simulink model "exampleModel_bus_axi_w_4ptavg"  (R2017b)
settings: Solver=VariableStepAuto  StartTime=0.0  StopTime=10e-5  RelTol=1e-3
PreLoadFcn:
  | setup
values from neighbouring files (symbols this model uses):
  axiClk = 156.25e6    (= 156250000)    [setup.m]    (also in setup_exampleModel_bus_axi_simulink.m; setup_exampleModel_bus_axi_simulink_lcls2.m; setup_lcls2_pcav.m; sysgen_signal.m)
  cav1p1_addr = 204    [setup_exampleModel_bus_axi_simulink.m]    (also in setup_exampleModel_bus_axi_simulink_lcls2.m; setup_lcls2_pcav.m; sysgen_signal.m)
  cav1p2_addr = cav1p1_addr * 2    (= 408)    [setup_exampleModel_bus_axi_simulink.m]    (also in setup_exampleModel_bus_axi_simulink_lcls2.m; setup_lcls2_pcav.m; sysgen_signal.m)
  cav2p1_addr = cav1p1_addr * 3    (= 612)    [setup_exampleModel_bus_axi_simulink.m]    (also in setup_exampleModel_bus_axi_simulink_lcls2.m; setup_lcls2_pcav.m; sysgen_signal.m)
  cav2p2_addr = cav1p1_addr * 4    (= 816)    [setup_exampleModel_bus_axi_simulink.m]    (also in setup_exampleModel_bus_axi_simulink_lcls2.m; setup_lcls2_pcav.m; sysgen_signal.m)
  Fadc = Fs/interleavedChannels    (= 29750000)    [setup.m]    (also in setup_exampleModel_bus_axi_simulink.m = 357000000; setup_exampleModel_bus_axi_simulink_lcls2.m = 351000000; setup_lcls2_pcav.m = 357000000; sysgen_signal.m = 357000000)
  fir_lpf = fir1(15, w_lpf)    [setup_exampleModel_bus_axi_simulink.m]    (also in setup_exampleModel_bus_axi_simulink_lcls2.m; setup_lcls2_pcav.m)
  Fproc = 204e6    (= 204000000)    [setup_exampleModel_bus_axi_simulink.m]    (also in setup_exampleModel_bus_axi_simulink_lcls2.m = 200571400; setup_lcls2_pcav.m; sysgen_signal.m)
  Fsig = Fproc/12    (= 17000000)    [setup_exampleModel_bus_axi_simulink.m]    (also in setup_exampleModel_bus_axi_simulink_lcls2.m = 16714283.3333; setup_lcls2_pcav.m)
  Tadc = 1/fadc    (= 2.80112044818e-09)    [cavity_signal.m]    (also in setup_exampleModel_bus_axi_simulink.m; setup_exampleModel_bus_axi_simulink_lcls2.m = 2.849002849e-09; setup_lcls2_pcav.m; setup_pcav_simulink.m)
undefined symbols (not defined in the file or in its folder): AXI4, Lite
libraries: xbsIndex_r4 x2870, llrf_lib x10, simulink x3
(part 9 of 15)

== system exampleModel_bus_axi_w_4ptavg/example/dsp/Cav2/IQ_integration2 ==
  cav_windowed_imag : Inport
  cav_windowed_real : Inport  Port=2
  ref_windowed_i : Inport  Port=3
  ref_windowed_q : Inport  Port=4
  window_profile : Inport  Port=5
  Accumulator{,1..3} (4 alike) : xbsIndex_r4/Accumulator  operation=Add  n_bits=32  overflow=Wrap  scale=1  rst=on  hasbypass=off  infoeditControl=reset for floating point data type must be asserted for a minimum of 2 cycles  en=off  latency=1  msb_inp=100  msb=100  lsb=-100  use_behavioral_HDL=on  implementation=Fabric  dbl_ovrd=off  block_type=accum
  Convert{1,3,5..6} (4 alike) : xbsIndex_r4/Convert  gui_display_data_type=Boolean  arith_type=Boolean  n_bits=16  bin_pt=14  float_type=Single  exp_bits=8  fraction_bits=24  quantization=Truncate  overflow=Wrap  en=off  latency=1  pipeline=off  dbl_ovrd=off  block_type=convert
  Convert{2,4,9..10} (4 alike) : xbsIndex_r4/Convert  gui_display_data_type=Fixed-point  arith_type="Signed  (2's comp)"  n_bits=20  bin_pt=18  float_type=Single  exp_bits=8  fraction_bits=24  quantization=Truncate  overflow=Wrap  en=off  latency=1  pipeline=off  dbl_ovrd=off  block_type=convert
  Display{1..8} (8 alike) : Display
  Gateway Out{,1..18,22..23} (21 alike) : xbsIndex_r4/Gateway Out  inherit_from_input=off  hdl_port=on  rows=1  columns=1  UseAsDAC=off  DACChannel='1'  interface=None  automatic_assignment=on  address_offset=hex2dec('00')  intf_name=''  intf_description=''  timing_constraint=None  locs_specified=off  LOCs={}  io_standard={}  block_type=gatewayout
  Inverter{,1..3} (4 alike) : xbsIndex_r4/Inverter  en=off  latency=1  dbl_ovrd=off  block_type=inv
  Register{1..2,11..12} (4 alike) : xbsIndex_r4/Register  init=0  rst=off  en=on  dbl_ovrd=off  block_type=register
  Scope{1..9} (9 alike) : Scope  NumInputPorts=3
  cav_int_q : Outport
  cav_int_i : Outport  Port=2
  ref_int_i : Outport  Port=3
  ref_int_q : Outport  Port=4
  wires:
  Gateway Out13/1 -> Display2/1, Scope6/2
  Gateway Out6/1 -> Scope3/3, Scope7/3
  Accumulator1/1 -> Register11/1, Gateway Out7/1
  cav_windowed_real/1 -> Accumulator1/1, Gateway Out8/1
  Gateway Out/1 -> Scope6/3, Scope2/3
  Convert6/1 -> Register11/2, Inverter1/1
  [window] -> Convert5/1
  Convert5/1 -> Register12/2, Inverter/1
  Gateway Out8/1 -> Scope3/1, Scope7/1
  Accumulator/1 -> Register12/1, Gateway Out3/1
  Gateway Out9/1 -> Display1/1, Scope7/2
  Gateway Out3/1 -> Scope2/2
  Gateway Out5/1 -> Scope6/1, Scope2/1
  [window] -> Convert6/1
  Inverter/1 -> Gateway Out/1, Accumulator/2
  cav_windowed_imag/1 -> Gateway Out5/1, Accumulator/1
  Gateway Out7/1 -> Scope3/2
  Gateway Out23/1 -> Display4/1
  Gateway Out22/1 -> Display3/1
  Inverter1/1 -> Accumulator1/2, Gateway Out6/1
  Inverter2/1 -> Gateway Out2/1, Accumulator2/2
  Gateway Out1/1 -> Scope9/3, Display6/1
  Gateway Out4/1 -> Scope1/2
  [window] -> Convert1/1
  Gateway Out11/1 -> Scope9/1, Scope4/2, Display5/1
  Gateway Out10/1 -> Scope4/1, Scope1/1
  Convert1/1 -> Register1/2, Inverter2/1
  ref_windowed_i/1 -> Gateway Out10/1, Accumulator2/1
  Accumulator2/1 -> Gateway Out4/1, Register1/1
  Gateway Out2/1 -> Scope4/3, Scope1/3
  Gateway Out16/1 -> Scope5/3, Scope8/3
  Accumulator3/1 -> Register2/1, Gateway Out17/1
  ref_windowed_q/1 -> Accumulator3/1, Gateway Out14/1
  Convert3/1 -> Register2/2, Inverter3/1
  Gateway Out14/1 -> Scope5/1, Scope8/1
  Gateway Out15/1 -> Display7/1, Scope8/2
  [window] -> Convert3/1
  Gateway Out17/1 -> Scope5/2
  Gateway Out12/1 -> Display8/1
  Inverter3/1 -> Accumulator3/2, Gateway Out16/1
  Convert9/1 -> Gateway Out22/1, cav_int_i/1
  Convert10/1 -> cav_int_q/1, Gateway Out23/1
  Convert2/1 -> ref_int_i/1, Gateway Out1/1
  Convert4/1 -> ref_int_q/1, Gateway Out12/1
  window_profile/1 -> [window]
  Register1/1 -> Gateway Out18/1, Convert2/1, Gateway Out11/1
  Gateway Out18/1 -> Scope9/2
  Register2/1 -> Convert4/1, Gateway Out15/1
  Register11/1 -> Convert9/1, Gateway Out9/1
  Register12/1 -> Convert10/1, Gateway Out13/1

== system exampleModel_bus_axi_w_4ptavg/example/dsp/Cav2/Masking_n_delay ==
  note: delay for the comparison because Axilite register
      | takes a about 40 dsp clk cycles to load in
  phi_reset_trig : Inport
  start_pt : Inport  Port=2
  stop_pt : Inport  Port=3
  delay_amt : Inport  Port=4
  delay_latch : Inport  Port=5
  AddSub1 : xbsIndex_r4/AddSub  mode=Addition  use_carryin=off  use_carryout=off  en=off  latency=1  precision=User Defined  arith_type=Unsigned  n_bits=16  bin_pt=0  quantization=Truncate  overflow=Wrap  use_behavioral_HDL=off  hw_selection=Fabric  pipelined=off  dbl_ovrd=off  block_type=addsub
  AddSub4 : xbsIndex_r4/AddSub  mode=Addition  use_carryin=off  use_carryout=off  en=on  latency=1  precision=User Defined  arith_type=Unsigned  n_bits=16  bin_pt=0  quantization=Truncate  overflow=Saturate  use_behavioral_HDL=off  hw_selection=Fabric  pipelined=off  dbl_ovrd=off  block_type=addsub
  Constant1 : xbsIndex_r4/Constant  const=0  gui_display_data_type=Fixed-point  arith_type=Unsigned  n_bits=16  bin_pt=0  preci_type=Single  exp_width=8  frac_width=24  explicit_period=off  period=1  equ=P=C  opselect=C  inp2=PCIN>>17  opr=+  inp1=P  carry=CIN  dbl_ovrd=off  block_type=constant
  Constant11 : xbsIndex_r4/Constant  const=55  gui_display_data_type=Fixed-point  arith_type=Unsigned  n_bits=16  bin_pt=0  preci_type=Single  exp_width=8  frac_width=24  explicit_period=off  period=1  equ=P=C  opselect=C  inp2=PCIN>>17  opr=+  inp1=P  carry=CIN  dbl_ovrd=off  block_type=constant
  Constant2 : xbsIndex_r4/Constant  const=84  gui_display_data_type=Fixed-point  arith_type=Unsigned  n_bits=16  bin_pt=0  preci_type=Single  exp_width=8  frac_width=24  explicit_period=off  period=1  equ=P=C  opselect=C  inp2=PCIN>>17  opr=+  inp1=P  carry=CIN  dbl_ovrd=off  block_type=constant
  Constant3 : xbsIndex_r4/Constant  const=62  gui_display_data_type=Fixed-point  arith_type=Unsigned  n_bits=16  bin_pt=0  preci_type=Single  exp_width=8  frac_width=24  explicit_period=off  period=1  equ=P=C  opselect=C  inp2=PCIN>>17  opr=+  inp1=P  carry=CIN  dbl_ovrd=off  block_type=constant
  Constant4 : xbsIndex_r4/Constant  const=0  gui_display_data_type=Fixed-point  arith_type=Unsigned  n_bits=1  bin_pt=0  preci_type=Single  exp_width=8  frac_width=24  explicit_period=off  period=1  equ=P=C  opselect=C  inp2=PCIN>>17  opr=+  inp1=P  carry=CIN  dbl_ovrd=off  block_type=constant
  Convert1 : xbsIndex_r4/Convert  gui_display_data_type=Fixed-point  arith_type=Unsigned  n_bits=8  bin_pt=0  float_type=Single  exp_bits=8  fraction_bits=24  quantization=Truncate  overflow=Saturate  en=off  latency=1  pipeline=off  dbl_ovrd=off  block_type=convert
  Convert11 : xbsIndex_r4/Convert  gui_display_data_type=Fixed-point  arith_type=Unsigned  n_bits=1  bin_pt=0  float_type=Single  exp_bits=8  fraction_bits=24  quantization=Truncate  overflow=Wrap  en=off  latency=1  pipeline=off  dbl_ovrd=off  block_type=convert
  Convert2 : xbsIndex_r4/Convert  gui_display_data_type=Fixed-point  arith_type=Unsigned  n_bits=1  bin_pt=0  float_type=Single  exp_bits=8  fraction_bits=24  quantization=Truncate  overflow=Wrap  en=off  latency=1  pipeline=off  dbl_ovrd=off  block_type=convert
  Convert3 : xbsIndex_r4/Convert  gui_display_data_type=Boolean  arith_type=Boolean  n_bits=16  bin_pt=14  float_type=Single  exp_bits=8  fraction_bits=24  quantization=Truncate  overflow=Wrap  en=off  latency=1  pipeline=off  dbl_ovrd=off  block_type=convert
  Convert5 : xbsIndex_r4/Convert  gui_display_data_type=Boolean  arith_type=Boolean  n_bits=1  bin_pt=0  float_type=Single  exp_bits=8  fraction_bits=24  quantization=Truncate  overflow=Wrap  en=off  latency=1  pipeline=off  dbl_ovrd=off  block_type=convert
  Convert7 : xbsIndex_r4/Convert  gui_display_data_type=Boolean  arith_type=Boolean  n_bits=1  bin_pt=0  float_type=Single  exp_bits=8  fraction_bits=24  quantization=Truncate  overflow=Wrap  en=off  latency=1  pipeline=off  dbl_ovrd=off  block_type=convert
  Convert8 : xbsIndex_r4/Convert  gui_display_data_type=Boolean  arith_type=Boolean  n_bits=1  bin_pt=0  float_type=Single  exp_bits=8  fraction_bits=24  quantization=Truncate  overflow=Wrap  en=off  latency=1  pipeline=off  dbl_ovrd=off  block_type=convert
  Counter : xbsIndex_r4/Counter  cnt_type=Count Limited  cnt_to=(2^15)  operation=Up  start_count=0  cnt_by_val=1  arith_type=Unsigned  n_bits=16  bin_pt=0  load_pin=off  rst=on  en=on  explicit_period=on  period=12/Fproc  use_behavioral_HDL=off  implementation=Fabric  dbl_ovrd=off  block_type=counter
  Delay{,1..4,6..7} (7 alike) : xbsIndex_r4/Delay  rst=off  infoeditControl=Selection of Reset will increase slice count due to use of real FFs and instead of SRLs  en=off  latency=1  reg_retiming=off  dbl_ovrd=off  block_type=delay
  Delay5 : xbsIndex_r4/Delay  rst=off  infoeditControl=Selection of Reset will increase slice count due to use of real FFs and instead of SRLs  en=off  latency=3  reg_retiming=off  dbl_ovrd=off  block_type=delay
  Delay8 : xbsIndex_r4/Delay  rst=off  infoeditControl=Selection of Reset will increase slice count due to use of real FFs and instead of SRLs  en=off  latency=4  reg_retiming=off  dbl_ovrd=off  block_type=delay
  Display1 : Display
  Down Sample1 : xbsIndex_r4/Down Sample  sample_ratio=12  sample_phase="Last Value of Frame  (most efficient)"  en=off  rst=off  latency=1  dbl_ovrd=off  block_type=dsamp
  Down Sample2 : xbsIndex_r4/Down Sample  sample_ratio=12  sample_phase="Last Value of Frame  (most efficient)"  en=off  rst=off  latency=1  dbl_ovrd=off  block_type=dsamp
  Gateway Out{1..9,27..29} (12 alike) : xbsIndex_r4/Gateway Out  inherit_from_input=off  hdl_port=on  rows=1  columns=1  UseAsDAC=off  DACChannel='1'  interface=None  automatic_assignment=on  address_offset=hex2dec('00')  intf_name=''  intf_description=''  timing_constraint=None  locs_specified=off  LOCs={}  io_standard={}  block_type=gatewayout
  Gateway Out16 : xbsIndex_r4/Gateway Out  inherit_from_input=off  hdl_port=off  rows=1  columns=1  UseAsDAC=off  DACChannel='1'  interface=None  automatic_assignment=on  address_offset=hex2dec('00')  intf_name=''  intf_description=''  timing_constraint=None  locs_specified=off  LOCs={}  io_standard={}  block_type=gatewayout
  Gateway Out17 : xbsIndex_r4/Gateway Out  inherit_from_input=off  hdl_port=off  rows=1  columns=1  UseAsDAC=off  DACChannel='1'  interface=None  automatic_assignment=on  address_offset=hex2dec('00')  intf_name=''  intf_description=''  timing_constraint=None  locs_specified=off  LOCs={}  io_standard={}  block_type=gatewayout
  Gateway Out18 : xbsIndex_r4/Gateway Out  inherit_from_input=off  hdl_port=off  rows=1  columns=1  UseAsDAC=off  DACChannel='1'  interface=None  automatic_assignment=on  address_offset=hex2dec('00')  intf_name=''  intf_description=''  timing_constraint=None  locs_specified=off  LOCs={}  io_standard={}  block_type=gatewayout
  Logical1 : xbsIndex_r4/Logical  logical_function=AND  inputs=2  en=off  latency=1  precision=Full  arith_type=Unsigned  n_bits=16  bin_pt=0  align_bp=on  dbl_ovrd=off  block_type=logical
  Logical2 : xbsIndex_r4/Logical  logical_function=AND  inputs=2  en=off  latency=1  precision=Full  arith_type=Unsigned  n_bits=16  bin_pt=0  align_bp=on  dbl_ovrd=off  block_type=logical
  Register : xbsIndex_r4/Register  init=44  rst=off  en=on  dbl_ovrd=off  block_type=register
  Register1 : xbsIndex_r4/Register  init=0  rst=off  en=on  dbl_ovrd=off  block_type=register
  Register10 : xbsIndex_r4/Register  init=0  rst=off  en=off  dbl_ovrd=off  block_type=register
  Register5 : xbsIndex_r4/Register  init=0  rst=off  en=off  dbl_ovrd=off  block_type=register
  Register6 : xbsIndex_r4/Register  init=100  rst=off  en=off  dbl_ovrd=off  block_type=register
  Relational1 : xbsIndex_r4/Relational  mode=a<b  op_type=Bool  en=on  latency=1  dbl_ovrd=off  block_type=relational
  Relational2 : xbsIndex_r4/Relational  mode=a>b  op_type=Bool  en=off  latency=1  dbl_ovrd=off  block_type=relational
  Relational3 : xbsIndex_r4/Relational  mode=a<b  op_type=Bool  en=on  latency=1  dbl_ovrd=off  block_type=relational
  Relational4 : xbsIndex_r4/Relational  mode=a>b  op_type=Bool  en=on  latency=1  dbl_ovrd=off  block_type=relational
  Relational5 : xbsIndex_r4/Relational  mode=a<b  op_type=Bool  en=on  latency=1  dbl_ovrd=off  block_type=relational
  Relational6 : xbsIndex_r4/Relational  mode=a>b  op_type=Bool  en=on  latency=1  dbl_ovrd=off  block_type=relational
  Relational7 : xbsIndex_r4/Relational  mode=a>b  op_type=Bool  en=off  latency=1  dbl_ovrd=off  block_type=relational
  Scope{1,3,5,10} (4 alike) : Scope  NumInputPorts=3
  Scope2 : Scope  NumInputPorts=2
  Scope4 : Scope  NumInputPorts=2
  trig_reset : Outport
  counter : Outport  Port=2
  eval_window : Outport  Port=3
  integral_trig : Outport  Port=4
  flo_window : Outport  Port=5
  Stream_valid : Outport  Port=6
  delay_val : Outport  Port=7
  wires:
  Gateway Out5/1 -> Scope2/2
  start_pt/1 -> Register5/1
  phi_reset_trig/1 -> Register10/1
  Register5/1 -> Down Sample1/1
  stop_pt/1 -> Register6/1
  Register6/1 -> Down Sample2/1
  Convert3/1 -> Register1/2, Register1/1, Gateway Out6/1, trig_reset/1, Counter/1
  Delay2/1 -> Relational4/2
  Delay3/1 -> AddSub1/1, Gateway Out2/1, Relational3/2
  Constant1/1 -> Relational2/2
  Relational3/1 -> Gateway Out28/1, Convert7/1
  Relational4/1 -> Gateway Out27/1, Convert8/1
  Gateway Out28/1 -> Scope10/2
  Gateway Out29/1 -> Scope2/1, Scope10/3
  Gateway Out27/1 -> Scope10/1
  Logical1/1 -> Convert11/1
  Convert8/1 -> Logical1/1
  Convert7/1 -> Gateway Out3/1, Logical1/2
  Convert11/1 -> eval_window/1, Gateway Out29/1
  Convert5/1 -> integral_trig/1, Gateway Out5/1
  Relational5/1 -> Convert5/1
  Relational2/1 -> Relational6/3, Relational1/3, Relational5/3, Relational3/3, Relational4/3
  Constant11/1 -> AddSub1/2
  AddSub1/1 -> Relational5/2
  Down Sample1/1 -> Delay2/1
  Down Sample2/1 -> Delay3/1
  Gateway Out1/1 -> Scope1/1
  Gateway Out2/1 -> Scope1/2
  Gateway Out3/1 -> Scope1/3
  Delay1/1 -> Relational4/1
  Delay4/1 -> Relational3/1
  Delay5/1 -> Gateway Out1/1
  Delay7/1 -> Relational1/1
  Constant2/1 -> Relational1/2
  Logical2/1 -> Convert2/1
  Relational1/1 -> Logical2/2
  Convert2/1 -> Gateway Out8/1, flo_window/1
  Delay6/1 -> Relational6/1
  Constant3/1 -> Relational6/2
  Relational6/1 -> Logical2/1
  Constant4/1 -> Relational7/2
  Relational7/1 -> Stream_valid/1
  Gateway Out4/1 -> Scope3/2
  Gateway Out6/1 -> Scope3/1
  Register10/1 -> Convert3/1
  Register1/1 -> Counter/2, Gateway Out7/1
  Gateway Out7/1 -> Scope3/3
  Gateway Out16/1 -> Scope5/1, Display1/1
  delay_latch/1 -> Gateway Out18/1, Delay/1, AddSub4/3
  delay_amt/1 -> AddSub4/2, Gateway Out16/1
  AddSub4/1 -> Register/1
  Gateway Out17/1 -> Scope5/2
  Gateway Out18/1 -> Scope5/3
  Register/1 -> AddSub4/1, delay_val/1, Gateway Out17/1
  Delay/1 -> Register/2
  Gateway Out8/1 -> Scope4/2
  Gateway Out9/1 -> Scope4/1
  Delay8/1 -> Gateway Out9/1
  Counter/1 -> Convert1/1
  Convert1/1 -> Gateway Out4/1, Relational7/1, Delay8/1, Delay5/1, counter/1, Delay1/1, Delay4/1, Relational2/1, Delay6/1, Delay7/1, Relational5/1

== system exampleModel_bus_axi_w_4ptavg/example/dsp/Cav2/PA_conversion1 ==
  cav_int_q : Inport
  cav_int_i : Inport  Port=2
  ref_int_q : Inport  Port=3
  ref_int_i : Inport  Port=4
  integration_trig : Inport  Port=5
  cal_coefficient : Inport  Port=6
  AddSub : xbsIndex_r4/AddSub  mode=Subtraction  use_carryin=off  use_carryout=off  en=off  latency=1  precision=User Defined  arith_type="Signed  (2's comp)"  n_bits=18  bin_pt=15  quantization=Truncate  overflow=Wrap  use_behavioral_HDL=off  hw_selection=Fabric  pipelined=off  dbl_ovrd=off  block_type=addsub
  AddSub1 : xbsIndex_r4/AddSub  mode=Addition  use_carryin=off  use_carryout=off  en=off  latency=1  precision=User Defined  arith_type="Signed  (2's comp)"  n_bits=18  bin_pt=15  quantization=Truncate  overflow=Wrap  use_behavioral_HDL=off  hw_selection=Fabric  pipelined=off  dbl_ovrd=off  block_type=addsub
  CORDIC 6.0 1 : xbsIndex_r4/CORDIC 6.0   functional_selection=Translate  architectural_configuration=Parallel  pipelining_mode=Maximum  data_format=SignedFraction  phase_format=Scaled_Radians  input_width=20  output_width=18  round_mode=Truncate  iterations=0  precision=0  compensation_scaling=No_Scale_Compensation  coarse_rotation=on  aclken=off  aresetn=off  out_tready=off  cartesian_has_tuser=off  cartesian_has_tlast=off  cartesian_tuser_width=1  phase_has_tuser=off  phase_has_tlast=off  phase_tuser_width=1  out_tlast_behv=Null  flow_control=NonBlocking  optimize_goal=Resources  trim_axipin_name=on  simulation_type=hybrid_sim  simulation_model=sysgen:cordic_v6_0  data_path_portlist={'s_axis_cartesian_tdata_imag', 's_axis_cartesian_tdata_real', 's_axis_phase_tdata_phase', 'm_axis_dout_tdata_imag', 'm_axis_dout_tdata_real', 'm_axis_dout_tdata_phase','m_axis_dout_tdata'}  ip_name=CORDIC  ip_version=6.0  dsptool_ready=true  ipcore_usecache=true  ipcore_useipmodelcache=true  wrapper_available=true  port_translation_map={ 'aclken' => 'en', 'aresetn' => 'rst' }  block_type=cordic_v6_0
      settings: infoedit=CORDIC 6.0
  CORDIC 6.0 2 : xbsIndex_r4/CORDIC 6.0   functional_selection=Translate  architectural_configuration=Parallel  pipelining_mode=Maximum  data_format=SignedFraction  phase_format=Scaled_Radians  input_width=20  output_width=18  round_mode=Truncate  iterations=0  precision=0  compensation_scaling=No_Scale_Compensation  coarse_rotation=on  aclken=off  aresetn=off  out_tready=off  cartesian_has_tuser=off  cartesian_has_tlast=off  cartesian_tuser_width=1  phase_has_tuser=off  phase_has_tlast=off  phase_tuser_width=1  out_tlast_behv=Null  flow_control=NonBlocking  optimize_goal=Resources  trim_axipin_name=on  simulation_type=hybrid_sim  simulation_model=sysgen:cordic_v6_0  data_path_portlist={'s_axis_cartesian_tdata_imag', 's_axis_cartesian_tdata_real', 's_axis_phase_tdata_phase', 'm_axis_dout_tdata_imag', 'm_axis_dout_tdata_real', 'm_axis_dout_tdata_phase','m_axis_dout_tdata'}  ip_name=CORDIC  ip_version=6.0  dsptool_ready=true  ipcore_usecache=true  ipcore_useipmodelcache=true  wrapper_available=true  port_translation_map={ 'aclken' => 'en', 'aresetn' => 'rst' }  block_type=cordic_v6_0
      settings: infoedit=CORDIC 6.0
  Delay{,1..3} (4 alike) : xbsIndex_r4/Delay  rst=off  infoeditControl=Selection of Reset will increase slice count due to use of real FFs and instead of SRLs  en=off  latency=1  reg_retiming=off  dbl_ovrd=off  block_type=delay
  Gateway Out{1..5,9,13,20..22,30..31,33} (13 alike) : xbsIndex_r4/Gateway Out  inherit_from_input=off  hdl_port=off  rows=1  columns=1  UseAsDAC=off  DACChannel='1'  interface=None  automatic_assignment=on  address_offset=hex2dec('00')  intf_name=''  intf_description=''  timing_constraint=None  locs_specified=off  LOCs={}  io_standard={}  block_type=gatewayout
  Gateway Out{6..8,24..26} (6 alike) : xbsIndex_r4/Gateway Out  inherit_from_input=off  hdl_port=on  rows=1  columns=1  UseAsDAC=off  DACChannel='1'  interface=None  automatic_assignment=on  address_offset=hex2dec('00')  intf_name=''  intf_description=''  timing_constraint=None  locs_specified=off  LOCs={}  io_standard={}  block_type=gatewayout
  Inverter{1..4} (4 alike) : xbsIndex_r4/Inverter  en=off  latency=1  dbl_ovrd=off  block_type=inv
  Register{11..14} (4 alike) : xbsIndex_r4/Register  init=0  rst=off  en=on  dbl_ovrd=off  block_type=register
  Scope{1..3,6,8,14..15} (7 alike) : Scope  NumInputPorts=3
  phi_diff : Outport
  ref_phi_out : Outport  Port=2
  ref_amp_out : Outport  Port=3
  cav_phi_out : Outport  Port=4
  cav_amp_out : Outport  Port=5
  wires:
  CORDIC 6.0 2/3 -> Gateway Out5/1, Delay2/1
  Gateway Out8/1 -> Scope6/3
  CORDIC 6.0 1/1 -> Inverter2/1, Inverter3/1
  Gateway Out33/1 -> Scope15/1
  CORDIC 6.0 2/1 -> Inverter4/1, Inverter1/1
  Inverter2/1 -> Register13/2
  Gateway Out7/1 -> Scope6/2
  Gateway Out22/1 -> Scope3/1
  Inverter1/1 -> Register11/2
  CORDIC 6.0 1/3 -> Delay/1, Gateway Out21/1
  Gateway Out25/1 -> Scope8/2
  Gateway Out26/1 -> Scope8/3
  CORDIC 6.0 2/2 -> Gateway Out3/1, Delay3/1
  Inverter3/1 -> Gateway Out30/1, Register14/2
  [trig] -> Gateway Out24/1, CORDIC 6.0 1/1
  Gateway Out5/1 -> Scope2/3
  Gateway Out21/1 -> Scope14/3
  Gateway Out3/1 -> Scope2/2
  cav_int_q/1 -> Gateway Out25/1, CORDIC 6.0 1/2
  Gateway Out31/1 -> Scope15/2
  Gateway Out30/1 -> Scope15/3, Scope14/1
  ref_int_i/1 -> Gateway Out8/1, CORDIC 6.0 2/3
  Gateway Out20/1 -> Scope14/2
  Inverter4/1 -> Gateway Out9/1, Register12/2
  Gateway Out9/1 -> Scope2/1, Scope3/3
  Gateway Out13/1 -> Scope3/2
  Gateway Out24/1 -> Scope8/1
  CORDIC 6.0 1/2 -> Delay1/1, Gateway Out20/1
  Gateway Out6/1 -> Scope6/1
  cav_int_i/1 -> Gateway Out26/1, CORDIC 6.0 1/3
  ref_int_q/1 -> Gateway Out7/1, CORDIC 6.0 2/2
  Delay/1 -> Register14/1
  Delay1/1 -> Register13/1
  Delay2/1 -> Register12/1
  Delay3/1 -> Register11/1
  [ref_phi_out] -> AddSub/2, Gateway Out4/1
  AddSub/1 -> Gateway Out1/1, phi_diff/1
  Gateway Out1/1 -> Scope1/1
  Gateway Out2/1 -> Scope1/2
  Gateway Out4/1 -> Scope1/3
  [trig] -> Gateway Out6/1, CORDIC 6.0 2/1
  integration_trig/1 -> [trig]
  AddSub1/1 -> Gateway Out2/1, AddSub/1
  [cav_phi_out] -> AddSub1/1
  cal_coefficient/1 -> AddSub1/2
  Register11/1 -> [ref_phi_out], ref_phi_out/1, Gateway Out22/1
  Register12/1 -> ref_amp_out/1, Gateway Out13/1
  Register13/1 -> [cav_phi_out], cav_phi_out/1, Gateway Out33/1
  Register14/1 -> cav_amp_out/1, Gateway Out31/1

== system exampleModel_bus_axi_w_4ptavg/example/dsp/Cav2/PA_conversion2 ==
  cav_int_q : Inport
  cav_int_i : Inport  Port=2
  ref_int_q : Inport  Port=3
  ref_int_i : Inport  Port=4
  integration_trig : Inport  Port=5
  cal_coefficient : Inport  Port=6
  AddSub : xbsIndex_r4/AddSub  mode=Subtraction  use_carryin=off  use_carryout=off  en=off  latency=1  precision=User Defined  arith_type="Signed  (2's comp)"  n_bits=18  bin_pt=15  quantization=Truncate  overflow=Wrap  use_behavioral_HDL=off  hw_selection=Fabric  pipelined=off  dbl_ovrd=off  block_type=addsub
  AddSub1 : xbsIndex_r4/AddSub  mode=Addition  use_carryin=off  use_carryout=off  en=off  latency=1  precision=User Defined  arith_type="Signed  (2's comp)"  n_bits=18  bin_pt=15  quantization=Truncate  overflow=Wrap  use_behavioral_HDL=off  hw_selection=Fabric  pipelined=off  dbl_ovrd=off  block_type=addsub
  CORDIC 6.0 1 : xbsIndex_r4/CORDIC 6.0   functional_selection=Translate  architectural_configuration=Parallel  pipelining_mode=Maximum  data_format=SignedFraction  phase_format=Scaled_Radians  input_width=20  output_width=18  round_mode=Truncate  iterations=0  precision=0  compensation_scaling=No_Scale_Compensation  coarse_rotation=on  aclken=off  aresetn=off  out_tready=off  cartesian_has_tuser=off  cartesian_has_tlast=off  cartesian_tuser_width=1  phase_has_tuser=off  phase_has_tlast=off  phase_tuser_width=1  out_tlast_behv=Null  flow_control=NonBlocking  optimize_goal=Resources  trim_axipin_name=on  simulation_type=hybrid_sim  simulation_model=sysgen:cordic_v6_0  data_path_portlist={'s_axis_cartesian_tdata_imag', 's_axis_cartesian_tdata_real', 's_axis_phase_tdata_phase', 'm_axis_dout_tdata_imag', 'm_axis_dout_tdata_real', 'm_axis_dout_tdata_phase','m_axis_dout_tdata'}  ip_name=CORDIC  ip_version=6.0  dsptool_ready=true  ipcore_usecache=true  ipcore_useipmodelcache=true  wrapper_available=true  port_translation_map={ 'aclken' => 'en', 'aresetn' => 'rst' }  block_type=cordic_v6_0
      settings: infoedit=CORDIC 6.0
  CORDIC 6.0 2 : xbsIndex_r4/CORDIC 6.0   functional_selection=Translate  architectural_configuration=Parallel  pipelining_mode=Maximum  data_format=SignedFraction  phase_format=Scaled_Radians  input_width=20  output_width=18  round_mode=Truncate  iterations=0  precision=0  compensation_scaling=No_Scale_Compensation  coarse_rotation=on  aclken=off  aresetn=off  out_tready=off  cartesian_has_tuser=off  cartesian_has_tlast=off  cartesian_tuser_width=1  phase_has_tuser=off  phase_has_tlast=off  phase_tuser_width=1  out_tlast_behv=Null  flow_control=NonBlocking  optimize_goal=Resources  trim_axipin_name=on  simulation_type=hybrid_sim  simulation_model=sysgen:cordic_v6_0  data_path_portlist={'s_axis_cartesian_tdata_imag', 's_axis_cartesian_tdata_real', 's_axis_phase_tdata_phase', 'm_axis_dout_tdata_imag', 'm_axis_dout_tdata_real', 'm_axis_dout_tdata_phase','m_axis_dout_tdata'}  ip_name=CORDIC  ip_version=6.0  dsptool_ready=true  ipcore_usecache=true  ipcore_useipmodelcache=true  wrapper_available=true  port_translation_map={ 'aclken' => 'en', 'aresetn' => 'rst' }  block_type=cordic_v6_0
      settings: infoedit=CORDIC 6.0
  Delay{,1..3} (4 alike) : xbsIndex_r4/Delay  rst=off  infoeditControl=Selection of Reset will increase slice count due to use of real FFs and instead of SRLs  en=off  latency=1  reg_retiming=off  dbl_ovrd=off  block_type=delay
  Gateway Out{1..5,9,13,20..22,30..31,33} (13 alike) : xbsIndex_r4/Gateway Out  inherit_from_input=off  hdl_port=off  rows=1  columns=1  UseAsDAC=off  DACChannel='1'  interface=None  automatic_assignment=on  address_offset=hex2dec('00')  intf_name=''  intf_description=''  timing_constraint=None  locs_specified=off  LOCs={}  io_standard={}  block_type=gatewayout
  Gateway Out{6..8,24..26} (6 alike) : xbsIndex_r4/Gateway Out  inherit_from_input=off  hdl_port=on  rows=1  columns=1  UseAsDAC=off  DACChannel='1'  interface=None  automatic_assignment=on  address_offset=hex2dec('00')  intf_name=''  intf_description=''  timing_constraint=None  locs_specified=off  LOCs={}  io_standard={}  block_type=gatewayout
  Inverter{1..4} (4 alike) : xbsIndex_r4/Inverter  en=off  latency=1  dbl_ovrd=off  block_type=inv
  Register{11..14} (4 alike) : xbsIndex_r4/Register  init=0  rst=off  en=on  dbl_ovrd=off  block_type=register
  Scope{1..3,6,8,14..15} (7 alike) : Scope  NumInputPorts=3
  phi_diff : Outport
  ref_phi_out : Outport  Port=2
  ref_amp_out : Outport  Port=3
  cav_phi_out : Outport  Port=4
  cav_amp_out : Outport  Port=5
  wires:
  Register14/1 -> Gateway Out31/1, cav_amp_out/1
  Register13/1 -> Gateway Out33/1, cav_phi_out/1, [cav_phi_out]
  Register12/1 -> Gateway Out13/1, ref_amp_out/1
  Register11/1 -> Gateway Out22/1, ref_phi_out/1, [ref_phi_out]
  cal_coefficient/1 -> AddSub1/2
  [cav_phi_out] -> AddSub1/1
  AddSub1/1 -> AddSub/1, Gateway Out2/1
  integration_trig/1 -> [trig]
  [trig] -> CORDIC 6.0 2/1, Gateway Out6/1
  Gateway Out4/1 -> Scope1/3
  Gateway Out2/1 -> Scope1/2
  Gateway Out1/1 -> Scope1/1
  AddSub/1 -> phi_diff/1, Gateway Out1/1
  [ref_phi_out] -> Gateway Out4/1, AddSub/2
  Delay3/1 -> Register11/1
  Delay2/1 -> Register12/1
  Delay1/1 -> Register13/1
  Delay/1 -> Register14/1
  ref_int_q/1 -> CORDIC 6.0 2/2, Gateway Out7/1
  cav_int_i/1 -> CORDIC 6.0 1/3, Gateway Out26/1
  Gateway Out6/1 -> Scope6/1
  CORDIC 6.0 1/2 -> Gateway Out20/1, Delay1/1
  Gateway Out24/1 -> Scope8/1
  Gateway Out13/1 -> Scope3/2
  Gateway Out9/1 -> Scope3/3, Scope2/1
  Inverter4/1 -> Register12/2, Gateway Out9/1
  Gateway Out20/1 -> Scope14/2
  ref_int_i/1 -> CORDIC 6.0 2/3, Gateway Out8/1
  Gateway Out30/1 -> Scope14/1, Scope15/3
  Gateway Out31/1 -> Scope15/2
  cav_int_q/1 -> CORDIC 6.0 1/2, Gateway Out25/1
  Gateway Out3/1 -> Scope2/2
  Gateway Out21/1 -> Scope14/3
  Gateway Out5/1 -> Scope2/3
  [trig] -> CORDIC 6.0 1/1, Gateway Out24/1
  Inverter3/1 -> Register14/2, Gateway Out30/1
  CORDIC 6.0 2/2 -> Delay3/1, Gateway Out3/1
  Gateway Out26/1 -> Scope8/3
  Gateway Out25/1 -> Scope8/2
  CORDIC 6.0 1/3 -> Gateway Out21/1, Delay/1
  Inverter1/1 -> Register11/2
  Gateway Out22/1 -> Scope3/1
  Gateway Out7/1 -> Scope6/2
  Inverter2/1 -> Register13/2
  CORDIC 6.0 2/1 -> Inverter1/1, Inverter4/1
  Gateway Out33/1 -> Scope15/1
  CORDIC 6.0 1/1 -> Inverter3/1, Inverter2/1
  Gateway Out8/1 -> Scope6/3
  CORDIC 6.0 2/3 -> Delay2/1, Gateway Out5/1

== system exampleModel_bus_axi_w_4ptavg/example/dsp/Cav2/PA_select ==
  PA_bus : Inport
  PA_chan_sel : Inport  Port=2
  Bus Creator3 : BusCreator  Inputs=3
  Bus Selector : BusSelector  OutputSignals=amp,phase,sync
  Bus Selector1 : BusSelector  OutputSignals=amp,phase,sync,channel
  Channel Select1 : llrf_lib/Sysgen/Single Rate/Channel Select  SystemSampleTime=-1
      settings: SourceProductName=LLRF Library
  Amp : Outport
  Phase : Outport  Port=2
  sync : Outport  Port=3
  wires:
  PA_bus/1 -> Bus Selector1/1
  PA_chan_sel/1 -> Channel Select1/5
  Bus Creator3/1 -> Bus Selector/1
  Channel Select1/3 -> Bus Creator3/3  "sync"
  Channel Select1/2 -> Bus Creator3/2  "phase"
  Channel Select1/1 -> Bus Creator3/1  "amp"
  Bus Selector1/4 -> Channel Select1/4  "<channel>"
  Bus Selector1/3 -> Channel Select1/3  "<sync>"
  Bus Selector1/2 -> Channel Select1/2  "<phase>"
  Bus Selector1/1 -> Channel Select1/1  "<amp>"
  Bus Selector/1 -> Amp/1  "<amp>"
  Bus Selector/2 -> Phase/1  "<phase>"
  Bus Selector/3 -> sync/1  "<sync>"

== system exampleModel_bus_axi_w_4ptavg/example/dsp/Cav2/PA_select1 ==
  PA_bus : Inport
  PA_chan_sel : Inport  Port=2
  Bus Creator3 : BusCreator  Inputs=3
  Bus Selector : BusSelector  OutputSignals=amp,phase,sync
  Bus Selector1 : BusSelector  OutputSignals=amp,phase,sync,channel
  Channel Select1 : llrf_lib/Sysgen/Single Rate/Channel Select  SystemSampleTime=-1
      settings: SourceProductName=LLRF Library
  Amp : Outport
  Phase : Outport  Port=2
  sync : Outport  Port=3
  wires:
  Bus Selector/3 -> sync/1  "<sync>"
  Bus Selector/2 -> Phase/1  "<phase>"
  Bus Selector/1 -> Amp/1  "<amp>"
  Bus Selector1/1 -> Channel Select1/1  "<amp>"
  Bus Selector1/2 -> Channel Select1/2  "<phase>"
  Bus Selector1/3 -> Channel Select1/3  "<sync>"
  Bus Selector1/4 -> Channel Select1/4  "<channel>"
  Channel Select1/1 -> Bus Creator3/1  "amp"
  Channel Select1/2 -> Bus Creator3/2  "phase"
  Channel Select1/3 -> Bus Creator3/3  "sync"
  Bus Creator3/1 -> Bus Selector/1
  PA_chan_sel/1 -> Channel Select1/5
  PA_bus/1 -> Bus Selector1/1

== system exampleModel_bus_axi_w_4ptavg/example/dsp/Cav2/Subsystem1 ==
  IQ_stream_in : Inport
  IQ_chan_sel : Inport  Port=2
  Bus Creator5 : BusCreator  Inputs=3
  Bus Selector : BusSelector  OutputSignals=ddcI,ddcQ,sync
  Bus Selector3 : BusSelector  OutputSignals=ddcI,ddcQ,ddcSync,ddcChannel
  Channel Select3 : llrf_lib/Sysgen/Single Rate/Channel Select  SystemSampleTime=-1
      settings: SourceProductName=LLRF Library
  ddcI : Outport
  ddcQ : Outport  Port=2
  sync : Outport  Port=3
  wires:
  Bus Selector/3 -> sync/1  "<sync>"
  Bus Selector/2 -> ddcQ/1  "<ddcQ>"
  Bus Selector/1 -> ddcI/1  "<ddcI>"
  Bus Creator5/1 -> Bus Selector/1
  Bus Selector3/3 -> Channel Select3/3  "<ddcSync>"
  Bus Selector3/4 -> Channel Select3/4  "<ddcChannel>"
  Bus Selector3/1 -> Channel Select3/1  "<ddcI>"
  Channel Select3/2 -> Bus Creator5/2  "ddcQ"
  Channel Select3/1 -> Bus Creator5/1  "ddcI"
  Bus Selector3/2 -> Channel Select3/2  "<ddcQ>"
  Channel Select3/3 -> Bus Creator5/3  "sync"
  IQ_chan_sel/1 -> Channel Select3/5
  IQ_stream_in/1 -> Bus Selector3/1

== system exampleModel_bus_axi_w_4ptavg/example/dsp/Cav2/Subsystem10 ==
  d : Inport
  reset : Inport  Port=2
  cntr : Inport  Port=3
  threshold : Inport  Port=4
  Register11 : xbsIndex_r4/Register  init=0  rst=on  en=on  dbl_ovrd=off  block_type=register
  Relational4 : xbsIndex_r4/Relational  mode=a>b  op_type=Bool  en=off  latency=1  dbl_ovrd=off  block_type=relational
  posedge_pulse : Subsystem
  q : Outport
  wires:
  threshold/1 -> Relational4/2
  reset/1 -> Register11/2
  Relational4/1 -> posedge_pulse/1(In1)
  posedge_pulse/1(Out1) -> Register11/3
  Register11/1 -> q/1
  cntr/1 -> Relational4/1
  d/1 -> Register11/1

== system exampleModel_bus_axi_w_4ptavg/example/dsp/Cav2/Subsystem11 ==
  d : Inport
  reset : Inport  Port=2
  cntr : Inport  Port=3
  threshold : Inport  Port=4
  Register11 : xbsIndex_r4/Register  init=0  rst=on  en=on  dbl_ovrd=off  block_type=register
  Relational4 : xbsIndex_r4/Relational  mode=a>b  op_type=Bool  en=off  latency=1  dbl_ovrd=off  block_type=relational
  posedge_pulse : Subsystem
  q : Outport
  wires:
  threshold/1 -> Relational4/2
  reset/1 -> Register11/2
  Relational4/1 -> posedge_pulse/1(In1)
  posedge_pulse/1(Out1) -> Register11/3
  Register11/1 -> q/1
  cntr/1 -> Relational4/1
  d/1 -> Register11/1

== system exampleModel_bus_axi_w_4ptavg/example/dsp/Cav2/Subsystem12 ==
  d : Inport
  reset : Inport  Port=2
  cntr : Inport  Port=3
  threshold : Inport  Port=4
  Register11 : xbsIndex_r4/Register  init=0  rst=on  en=on  dbl_ovrd=off  block_type=register
  Relational4 : xbsIndex_r4/Relational  mode=a>b  op_type=Bool  en=off  latency=1  dbl_ovrd=off  block_type=relational
  posedge_pulse : Subsystem
  q : Outport
  wires:
  d/1 -> Register11/1
  cntr/1 -> Relational4/1
  Register11/1 -> q/1
  posedge_pulse/1(Out1) -> Register11/3
  Relational4/1 -> posedge_pulse/1(In1)
  reset/1 -> Register11/2
  threshold/1 -> Relational4/2

== system exampleModel_bus_axi_w_4ptavg/example/dsp/Cav2/Subsystem2 ==
  imag : Inport
  real : Inport  Port=2
  flo_window : Inport  Port=3
  reset : Inport  Port=4
  CORDIC 6.0 2 : xbsIndex_r4/CORDIC 6.0   functional_selection=Translate  architectural_configuration=Parallel  pipelining_mode=Maximum  data_format=SignedFraction  phase_format=Scaled_Radians  input_width=18  output_width=18  round_mode=Truncate  iterations=0  precision=0  compensation_scaling=No_Scale_Compensation  coarse_rotation=on  aclken=off  aresetn=off  out_tready=off  cartesian_has_tuser=off  cartesian_has_tlast=off  cartesian_tuser_width=1  phase_has_tuser=off  phase_has_tlast=off  phase_tuser_width=1  out_tlast_behv=Null  flow_control=NonBlocking  optimize_goal=Resources  trim_axipin_name=on  simulation_type=hybrid_sim  simulation_model=sysgen:cordic_v6_0  data_path_portlist={'s_axis_cartesian_tdata_imag', 's_axis_cartesian_tdata_real', 's_axis_phase_tdata_phase', 'm_axis_dout_tdata_imag', 'm_axis_dout_tdata_real', 'm_axis_dout_tdata_phase','m_axis_dout_tdata'}  ip_name=CORDIC  ip_version=6.0  dsptool_ready=true  ipcore_usecache=true  ipcore_useipmodelcache=true  wrapper_available=true  port_translation_map={ 'aclken' => 'en', 'aresetn' => 'rst' }  block_type=cordic_v6_0
      settings: infoedit=CORDIC 6.0
  Clock Enable Probe4 : xbsIndex_r4/Clock Enable Probe  inherit_constraints=on  block_type=ceprobe
      settings: infoedit="Clock enable extractor.  Produces a Boolean output that mirrors the hardware clock enable associated with the input sample rate.<br><br>Hardware notes: in hardware this block costs nothing."
  Down Sample5 : xbsIndex_r4/Down Sample  sample_ratio=12  sample_phase="Last Value of Frame  (most efficient)"  en=off  rst=off  latency=1  dbl_ovrd=off  block_type=dsamp
  Gateway Out{38,41,51..53} (5 alike) : xbsIndex_r4/Gateway Out  inherit_from_input=off  hdl_port=off  rows=1  columns=1  UseAsDAC=off  DACChannel='1'  interface=None  automatic_assignment=on  address_offset=hex2dec('00')  intf_name=''  intf_description=''  timing_constraint=None  locs_specified=off  LOCs={}  io_standard={}  block_type=gatewayout
  Gateway Out44 : xbsIndex_r4/Gateway Out  inherit_from_input=off  hdl_port=on  rows=1  columns=1  UseAsDAC=off  DACChannel='1'  interface=None  automatic_assignment=on  address_offset=hex2dec('00')  intf_name=''  intf_description=''  timing_constraint=None  locs_specified=off  LOCs={}  io_standard={}  block_type=gatewayout
  Gateway Out46 : xbsIndex_r4/Gateway Out  inherit_from_input=off  hdl_port=on  rows=1  columns=1  UseAsDAC=off  DACChannel='1'  interface=None  automatic_assignment=on  address_offset=hex2dec('00')  intf_name=''  intf_description=''  timing_constraint=None  locs_specified=off  LOCs={}  io_standard={}  block_type=gatewayout
  Scope20 : Scope  NumInputPorts=2
  Scope21 : Scope  NumInputPorts=3
  Scope22 : Scope  NumInputPorts=2
  four_point_avg1 : Subsystem
  freq_err1 : Subsystem
  NCO_err_fb : Outport
  freq_err : Outport  Port=2
  wires:
  [c1p2_pt_cntr] -> Gateway Out41/1
  Down Sample5/1 -> CORDIC 6.0 2/1
  Gateway Out51/1 -> Scope20/1
  Gateway Out38/1 -> Scope21/2
  reset/1 -> freq_err1/3(reset)
  CORDIC 6.0 2/3 -> four_point_avg1/1(In1), Gateway Out51/1, Gateway Out53/1
  Clock Enable Probe4/1 -> Down Sample5/1
  CORDIC 6.0 2/2 -> freq_err1/1(raw_phase), Gateway Out38/1
  four_point_avg1/1(Out1) -> Gateway Out52/1
  real/1 -> CORDIC 6.0 2/3, Gateway Out44/1
  imag/1 -> CORDIC 6.0 2/2, Clock Enable Probe4/1, Gateway Out46/1
  flo_window/1 -> freq_err1/2(window)
  Gateway Out44/1 -> Scope22/2
  Gateway Out53/1 -> Scope21/1
  Gateway Out41/1 -> Scope21/3
  freq_err1/1(NCO_err) -> NCO_err_fb/1
  Gateway Out46/1 -> Scope22/1
  Gateway Out52/1 -> Scope20/2
  freq_err1/2(freq_err) -> freq_err/1

== system exampleModel_bus_axi_w_4ptavg/example/dsp/Cav2/Subsystem3 ==
  IQ_stream_in : Inport
  IQ_chan_sel : Inport  Port=2
  Bus Creator5 : BusCreator  Inputs=3
  Bus Selector : BusSelector  OutputSignals=ddcI,ddcQ,sync
  Bus Selector3 : BusSelector  OutputSignals=ddcI,ddcQ,ddcSync,ddcChannel
  Channel Select3 : llrf_lib/Sysgen/Single Rate/Channel Select  SystemSampleTime=-1
      settings: SourceProductName=LLRF Library
  ddcI : Outport
  ddcQ : Outport  Port=2
  sync : Outport  Port=3
  wires:
  IQ_stream_in/1 -> Bus Selector3/1
  IQ_chan_sel/1 -> Channel Select3/5
  Channel Select3/3 -> Bus Creator5/3  "sync"
  Bus Selector3/2 -> Channel Select3/2  "<ddcQ>"
  Channel Select3/1 -> Bus Creator5/1  "ddcI"
  Channel Select3/2 -> Bus Creator5/2  "ddcQ"
  Bus Selector3/1 -> Channel Select3/1  "<ddcI>"
  Bus Selector3/4 -> Channel Select3/4  "<ddcChannel>"
  Bus Selector3/3 -> Channel Select3/3  "<ddcSync>"
  Bus Creator5/1 -> Bus Selector/1
  Bus Selector/1 -> ddcI/1  "<ddcI>"
  Bus Selector/2 -> ddcQ/1  "<ddcQ>"
  Bus Selector/3 -> sync/1  "<sync>"

== system exampleModel_bus_axi_w_4ptavg/example/dsp/Cav2/Subsystem4 ==
  imag : Inport
  real : Inport  Port=2
  flo_window : Inport  Port=3
  reset : Inport  Port=4
  CORDIC 6.0 2 : xbsIndex_r4/CORDIC 6.0   functional_selection=Translate  architectural_configuration=Parallel  pipelining_mode=Maximum  data_format=SignedFraction  phase_format=Scaled_Radians  input_width=18  output_width=18  round_mode=Truncate  iterations=0  precision=0  compensation_scaling=No_Scale_Compensation  coarse_rotation=on  aclken=off  aresetn=off  out_tready=off  cartesian_has_tuser=off  cartesian_has_tlast=off  cartesian_tuser_width=1  phase_has_tuser=off  phase_has_tlast=off  phase_tuser_width=1  out_tlast_behv=Null  flow_control=NonBlocking  optimize_goal=Resources  trim_axipin_name=on  simulation_type=hybrid_sim  simulation_model=sysgen:cordic_v6_0  data_path_portlist={'s_axis_cartesian_tdata_imag', 's_axis_cartesian_tdata_real', 's_axis_phase_tdata_phase', 'm_axis_dout_tdata_imag', 'm_axis_dout_tdata_real', 'm_axis_dout_tdata_phase','m_axis_dout_tdata'}  ip_name=CORDIC  ip_version=6.0  dsptool_ready=true  ipcore_usecache=true  ipcore_useipmodelcache=true  wrapper_available=true  port_translation_map={ 'aclken' => 'en', 'aresetn' => 'rst' }  block_type=cordic_v6_0
      settings: infoedit=CORDIC 6.0
  Clock Enable Probe4 : xbsIndex_r4/Clock Enable Probe  inherit_constraints=on  block_type=ceprobe
      settings: infoedit="Clock enable extractor.  Produces a Boolean output that mirrors the hardware clock enable associated with the input sample rate.<br><br>Hardware notes: in hardware this block costs nothing."
  Down Sample5 : xbsIndex_r4/Down Sample  sample_ratio=12  sample_phase="Last Value of Frame  (most efficient)"  en=off  rst=off  latency=1  dbl_ovrd=off  block_type=dsamp
  Gateway Out{1,38,41,51..53} (6 alike) : xbsIndex_r4/Gateway Out  inherit_from_input=off  hdl_port=off  rows=1  columns=1  UseAsDAC=off  DACChannel='1'  interface=None  automatic_assignment=on  address_offset=hex2dec('00')  intf_name=''  intf_description=''  timing_constraint=None  locs_specified=off  LOCs={}  io_standard={}  block_type=gatewayout
  Gateway Out44 : xbsIndex_r4/Gateway Out  inherit_from_input=off  hdl_port=on  rows=1  columns=1  UseAsDAC=off  DACChannel='1'  interface=None  automatic_assignment=on  address_offset=hex2dec('00')  intf_name=''  intf_description=''  timing_constraint=None  locs_specified=off  LOCs={}  io_standard={}  block_type=gatewayout
  Gateway Out46 : xbsIndex_r4/Gateway Out  inherit_from_input=off  hdl_port=on  rows=1  columns=1  UseAsDAC=off  DACChannel='1'  interface=None  automatic_assignment=on  address_offset=hex2dec('00')  intf_name=''  intf_description=''  timing_constraint=None  locs_specified=off  LOCs={}  io_standard={}  block_type=gatewayout
  Scope20 : Scope  NumInputPorts=2
  Scope21 : Scope  NumInputPorts=4
  Scope22 : Scope  NumInputPorts=2
  four_point_avg1 : Subsystem
  freq_err1 : Subsystem
  NCO_err_fb : Outport
  freq_err : Outport  Port=2
  wires:
  [c1p2_pt_cntr] -> Gateway Out41/1
  Down Sample5/1 -> CORDIC 6.0 2/1
  Gateway Out51/1 -> Scope20/1
  Gateway Out38/1 -> Scope21/2
  reset/1 -> freq_err1/3(reset)
  CORDIC 6.0 2/3 -> four_point_avg1/1(In1), Gateway Out51/1, Gateway Out53/1
  Clock Enable Probe4/1 -> Down Sample5/1
  CORDIC 6.0 2/2 -> freq_err1/1(raw_phase), Gateway Out38/1
  four_point_avg1/1(Out1) -> Gateway Out52/1
  real/1 -> CORDIC 6.0 2/3, Gateway Out44/1
  imag/1 -> CORDIC 6.0 2/2, Clock Enable Probe4/1, Gateway Out46/1
  flo_window/1 -> Gateway Out1/1, freq_err1/2(window)
  Gateway Out44/1 -> Scope22/2
  Gateway Out53/1 -> Scope21/1
  Gateway Out41/1 -> Scope21/3
  freq_err1/1(NCO_err) -> NCO_err_fb/1
  Gateway Out46/1 -> Scope22/1
  Gateway Out52/1 -> Scope20/2
  freq_err1/2(freq_err) -> freq_err/1
  Gateway Out1/1 -> Scope21/4

== system exampleModel_bus_axi_w_4ptavg/example/dsp/Cav2/Subsystem5 ==
  d : Inport
  reset : Inport  Port=2
  cntr : Inport  Port=3
  threshold : Inport  Port=4
  Register11 : xbsIndex_r4/Register  init=0  rst=on  en=on  dbl_ovrd=off  block_type=register
  Relational4 : xbsIndex_r4/Relational  mode=a>b  op_type=Bool  en=off  latency=1  dbl_ovrd=off  block_type=relational
  posedge_pulse : Subsystem
  q : Outport
  wires:
  d/1 -> Register11/1
  cntr/1 -> Relational4/1
  Register11/1 -> q/1
  posedge_pulse/1(Out1) -> Register11/3
  Relational4/1 -> posedge_pulse/1(In1)
  reset/1 -> Register11/2
  threshold/1 -> Relational4/2

== system exampleModel_bus_axi_w_4ptavg/example/dsp/Cav2/Subsystem6 ==
  d : Inport
  reset : Inport  Port=2
  cntr : Inport  Port=3
  threshold : Inport  Port=4
  Register11 : xbsIndex_r4/Register  init=0  rst=on  en=on  dbl_ovrd=off  block_type=register
  Relational4 : xbsIndex_r4/Relational  mode=a>b  op_type=Bool  en=off  latency=1  dbl_ovrd=off  block_type=relational
  posedge_pulse : Subsystem
  q : Outport
  wires:
  threshold/1 -> Relational4/2
  reset/1 -> Register11/2
  Relational4/1 -> posedge_pulse/1(In1)
  posedge_pulse/1(Out1) -> Register11/3
  Register11/1 -> q/1
  cntr/1 -> Relational4/1
  d/1 -> Register11/1

== system exampleModel_bus_axi_w_4ptavg/example/dsp/Cav2/Subsystem7 ==
  d : Inport
  reset : Inport  Port=2
  cntr : Inport  Port=3
  threshold : Inport  Port=4
  Register11 : xbsIndex_r4/Register  init=0  rst=on  en=on  dbl_ovrd=off  block_type=register
  Relational4 : xbsIndex_r4/Relational  mode=a>b  op_type=Bool  en=off  latency=1  dbl_ovrd=off  block_type=relational
  posedge_pulse : Subsystem
  q : Outport
  wires:
  d/1 -> Register11/1
  cntr/1 -> Relational4/1
  Register11/1 -> q/1
  posedge_pulse/1(Out1) -> Register11/3
  Relational4/1 -> posedge_pulse/1(In1)
  reset/1 -> Register11/2
  threshold/1 -> Relational4/2

== system exampleModel_bus_axi_w_4ptavg/example/dsp/Cav2/Subsystem8 ==
  d : Inport
  reset : Inport  Port=2
  cntr : Inport  Port=3
  threshold : Inport  Port=4
  Register11 : xbsIndex_r4/Register  init=0  rst=on  en=on  dbl_ovrd=off  block_type=register
  Relational4 : xbsIndex_r4/Relational  mode=a>b  op_type=Bool  en=off  latency=1  dbl_ovrd=off  block_type=relational
  posedge_pulse : Subsystem
  q : Outport
  wires:
  threshold/1 -> Relational4/2
  reset/1 -> Register11/2
  Relational4/1 -> posedge_pulse/1(In1)
  posedge_pulse/1(Out1) -> Register11/3
  Register11/1 -> q/1
  cntr/1 -> Relational4/1
  d/1 -> Register11/1

== system exampleModel_bus_axi_w_4ptavg/example/dsp/Cav2/Subsystem9 ==
  d : Inport
  reset : Inport  Port=2
  cntr : Inport  Port=3
  threshold : Inport  Port=4
  Register11 : xbsIndex_r4/Register  init=0  rst=on  en=on  dbl_ovrd=off  block_type=register
  Relational4 : xbsIndex_r4/Relational  mode=a>b  op_type=Bool  en=off  latency=1  dbl_ovrd=off  block_type=relational
  posedge_pulse : Subsystem
  q : Outport
  wires:
  d/1 -> Register11/1
  cntr/1 -> Relational4/1
  Register11/1 -> q/1
  posedge_pulse/1(Out1) -> Register11/3
  Relational4/1 -> posedge_pulse/1(In1)
  reset/1 -> Register11/2
  threshold/1 -> Relational4/2

== system exampleModel_bus_axi_w_4ptavg/example/dsp/Cav2/c1p2_windowing_func2 ==
  imag : Inport
  real : Inport  Port=2
  eval_window : Inport  Port=3
  "CORDIC 6.0 " : xbsIndex_r4/CORDIC 6.0   functional_selection=Translate  architectural_configuration=Parallel  pipelining_mode=Maximum  data_format=SignedFraction  phase_format=Scaled_Radians  input_width=18  output_width=18  round_mode=Truncate  iterations=0  precision=0  compensation_scaling=No_Scale_Compensation  coarse_rotation=on  aclken=off  aresetn=off  out_tready=off  cartesian_has_tuser=off  cartesian_has_tlast=off  cartesian_tuser_width=1  phase_has_tuser=off  phase_has_tlast=off  phase_tuser_width=1  out_tlast_behv=Null  flow_control=NonBlocking  optimize_goal=Resources  trim_axipin_name=on  simulation_type=hybrid_sim  simulation_model=sysgen:cordic_v6_0  data_path_portlist={'s_axis_cartesian_tdata_imag', 's_axis_cartesian_tdata_real', 's_axis_phase_tdata_phase', 'm_axis_dout_tdata_imag', 'm_axis_dout_tdata_real', 'm_axis_dout_tdata_phase','m_axis_dout_tdata'}  ip_name=CORDIC  ip_version=6.0  dsptool_ready=true  ipcore_usecache=true  ipcore_useipmodelcache=true  wrapper_available=true  port_translation_map={ 'aclken' => 'en', 'aresetn' => 'rst' }  block_type=cordic_v6_0
      settings: infoedit=CORDIC 6.0
  Gateway Out{1..5,7} (6 alike) : xbsIndex_r4/Gateway Out  inherit_from_input=off  hdl_port=off  rows=1  columns=1  UseAsDAC=off  DACChannel='1'  interface=None  automatic_assignment=on  address_offset=hex2dec('00')  intf_name=''  intf_description=''  timing_constraint=None  locs_specified=off  LOCs={}  io_standard={}  block_type=gatewayout
  Scope{1..4} (4 alike) : Scope  NumInputPorts=3
  four_point_avg : Subsystem
  Window_profile : Outport
  wires:
  Gateway Out3/1 -> Scope4/3
  [window] -> Gateway Out3/1
  Gateway Out2/1 -> Scope1/2
  Gateway Out1/1 -> Scope1/1
  Gateway Out4/1 -> Scope2/1, Scope4/1
  "CORDIC 6.0 "/2 -> Gateway Out5/1
  eval_window/1 -> [window]
  [c1p2_pt_cntr] -> Gateway Out7/1
  Gateway Out7/1 -> Scope3/2, Scope4/2
  Gateway Out5/1 -> Scope2/2, Scope3/1
  real/1 -> "CORDIC 6.0 "/3
  imag/1 -> "CORDIC 6.0 "/2
  [cav1_p2_dc_tvalid] -> "CORDIC 6.0 "/1
  "CORDIC 6.0 "/3 -> four_point_avg/1(In1), Gateway Out1/1, Gateway Out4/1
  four_point_avg/1(Out1) -> Window_profile/1, Gateway Out2/1
